simulink model "test02"  (R2025b)
settings: Solver=VariableStepAuto  StartTime=0.0  StopTime=10.0  RelTol=1e-3
settings Model: Creator=sanborkl  LastModifiedBy=sanborkl

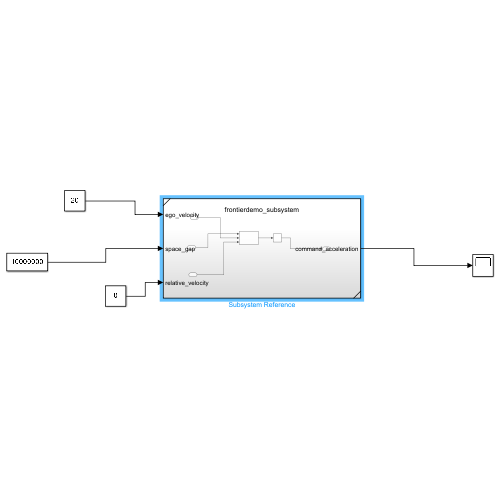
[thumbnail: Simulink's stored preview of the top-level diagram]
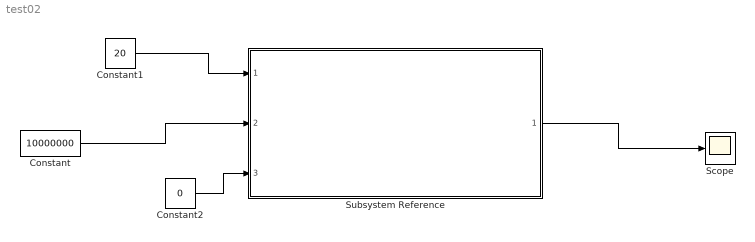
== system test02 ==
  Constant : Constant  Value=10000000
  Constant1 : Constant  Value=20
  Constant2 : Constant  Value=0
  Scope : Scope
      settings: ActiveDisplayYMinimum=-1  ActiveDisplayYMaximum=1
  Subsystem Reference : Subsystem  ReferencedSubsystem=frontierdemo_subsystem
  wires:
  Constant1/1 -> Subsystem Reference/1
  Constant/1 -> Subsystem Reference/2
  Subsystem Reference/1 -> Scope/1
  Constant2/1 -> Subsystem Reference/3
